simulink model "D_20231120_Modell_Inbetriebnahme_BreakOutBox_Jetson"  (R2022b)
settings: Solver=ode1  StartTime=0.0  StopTime=inf  FixedStep=Ts  RelTol=1e-3
PreLoadFcn:
  | pulsePeriod = 0.05;
  | 
  | Ts = 0.001;
  | 
  | FPGA_Frequency = 75000000;
  | 
  | ts_IO691 = 5e-3;
PostLoadFcn:
  | ewolfSetUp
InitFcn:
  | pulsePeriod = 0.05;
  | 
  | Ts = 0.001;
  | 
  | FPGA_Frequency = 75000000;
  | 
  | ts_IO691 = 5e-3;
StopFcn:
  | Simulink.sdi.clearPreferences;
  | if isfile(['sdi_view_',bdroot,'.mldatx'])
  | Simulink.sdi.view;
  | pause(3);
  | Simulink.sdi.loadView(['sdi_view_',bdroot,]);
  | end
model workspace (MAT data in the model file):
  MaxDreh = 1
values from neighbouring files (symbols this model uses):
  max_ac = 2    [ewolfSetUp.m]
  min_ac = -3    [ewolfSetUp.m]
  PredictionHorizon = 30    [ewolfSetUp.m]
undefined symbols (not defined in the file or in its folder): canChannel, DiscIntNeverNeededParam, Ended, HS, IO291, IO397, max_steer_car, min_steer_car, sigbuilder_block, Single
libraries: lllalib x255, canmsglib x146, simulink x42, speedgoatlib_IO191 x5, speedgoatlib_IO291 x5, slrealtimeiplib x3, speedgoatlib_IO691 x3, slrealtimeutilitieslib x2, spsEdgeDetectorLib x1, simulink_extras x1, speedgoatlib_fpga_dio x1, speedgoatlib_fpga_quadrature x1
(part 2 of 8)

== system D_20231120_Modell_Inbetriebnahme_BreakOutBox_Jetson/Scope ==
  From_Speedgoat : Inport
  To_Speedgoat : Inport  Port=2
  Bus Selector : BusSelector  OutputSignals=IO191_Out.IO191_AI.IO191_AI_CH1_FP_1_G,IO191_Out.IO191_AI.IO191_AI_CH2_FP_2_G,IO191_Out.IO191_AI.IO191_AI_CH3_LG_1_G,IO191_Out.IO191_AI.IO191_AI_CH4_LG_2_G
  Bus Selector1 : BusSelector  OutputSignals=IO691_Out.IO691_CAN_Sensoren.USS,IO691_Out.IO691_CAN_Sensoren.RC_Lenkung,IO691_Out.IO691_CAN_Sensoren.RC_Fahrpedal
  Scope : Scope  NumInputPorts=3
  Scope2 : Scope  NumInputPorts=4
  Terminator : Terminator
  wires:
  Bus Selector/2 -> Scope2/2  "<IO191_AI_CH2_FP_2_G>"
  Bus Selector/1 -> Scope2/1  "<IO191_AI_CH1_FP_1_G>"
  Bus Selector/4 -> Scope2/4  "<IO191_AI_CH4_LG_2_G>"
  From_Speedgoat/1 -> Bus Selector1/1, Bus Selector/1
  Bus Selector/3 -> Scope2/3  "<IO191_AI_CH3_LG_1_G>"
  To_Speedgoat/1 -> Terminator/1
  Bus Selector1/1 -> Scope/1  "<USS>"
  Bus Selector1/2 -> Scope/2  "<RC_Lenkung>"
  Bus Selector1/3 -> Scope/3  "<RC_Fahrpedal>"

== system D_20231120_Modell_Inbetriebnahme_BreakOutBox_Jetson/Bremspedal Steuerung/Moving Average ==
  In : Inport
  Divide : Product  Inputs=*/
  Round : Rounding  Operator=round
  Sum of Elements : Sum  Inputs=+
  Tapped Delay : simulink/Discrete/Tapped Delay  vinit=0.0  samptime=-1  NumDelays=4  DelayOrder=Oldest  includeCurrent=off
  Vector Concatenate : Concatenate
  Width : Width
  Hall_A : Outport
  wires:
  In/1 -> Vector Concatenate/1, Tapped Delay/1
  Sum of Elements/1 -> Divide/1
  Width/1 -> Divide/2
  Vector Concatenate/1 -> Sum of Elements/1, Width/1
  Divide/1 -> Round/1
  Round/1 -> Hall_A/1
  Tapped Delay/1 -> Vector Concatenate/2

== system D_20231120_Modell_Inbetriebnahme_BreakOutBox_Jetson/Bremspedal Steuerung/Moving Average1 ==
  In : Inport
  Divide : Product  Inputs=*/
  Round : Rounding  Operator=round
  Sum of Elements : Sum  Inputs=+
  Tapped Delay : simulink/Discrete/Tapped Delay  vinit=0.0  samptime=-1  NumDelays=4  DelayOrder=Oldest  includeCurrent=off
  Vector Concatenate : Concatenate
  Width : Width
  Hall_B : Outport
  wires:
  In/1 -> Vector Concatenate/1, Tapped Delay/1
  Sum of Elements/1 -> Divide/1
  Width/1 -> Divide/2
  Vector Concatenate/1 -> Sum of Elements/1, Width/1
  Divide/1 -> Round/1
  Round/1 -> Hall_B/1
  Tapped Delay/1 -> Vector Concatenate/2

== system D_20231120_Modell_Inbetriebnahme_BreakOutBox_Jetson/Bremspedal Steuerung/QAD Steuerung ==
  <QAD_Turns> : Inport
  u : Inport  Port=2
  AND : Logic  Inputs=3  AllPortsSameDT=off  OutDataTypeStr=boolean
  AND1 : Logic  AllPortsSameDT=off  OutDataTypeStr=boolean
  AND2 : Logic  AllPortsSameDT=off  OutDataTypeStr=boolean
  Compare To Constant : simulink/Logic and Bit Operations/Compare To Constant  relop=>  const=0.4  OutDataTypeStr=boolean
  Compare To Constant1 : simulink/Logic and Bit Operations/Compare To Constant  relop=<  const=0.1  OutDataTypeStr=boolean
  Compare To Constant2 : simulink/Logic and Bit Operations/Compare To Constant  relop=<  const=0  OutDataTypeStr=boolean
  Compare To Constant3 : simulink/Logic and Bit Operations/Compare To Constant  relop=>=  const=-0.2  OutDataTypeStr=boolean
  Compare To Constant4 : simulink/Logic and Bit Operations/Compare To Constant  relop=<  const=0.9  OutDataTypeStr=boolean
  Compare To Constant5 : simulink/Logic and Bit Operations/Compare To Constant  relop=>  const=0.9  OutDataTypeStr=boolean
  Compare To Constant6 : simulink/Logic and Bit Operations/Compare To Constant  relop=>=  const=-0.4  OutDataTypeStr=boolean
  IC2 : InitialCondition  Value=0
  IC3 : InitialCondition  Value=0
  OR : Logic  Operator=OR  AllPortsSameDT=off  OutDataTypeStr=boolean
  Out1 : Outport
  Out2 : Outport  Port=2
  wires:
  <QAD_Turns>/1 -> Compare To Constant3/1, Compare To Constant2/1, Compare To Constant6/1
  OR/1 -> IC2/1
  AND1/1 -> IC3/1
  IC3/1 -> Out2/1
  u/1 -> Compare To Constant5/1, Compare To Constant4/1, Compare To Constant/1, Compare To Constant1/1
  IC2/1 -> Out1/1
  Compare To Constant/1 -> AND/2
  Compare To Constant6/1 -> AND2/2
  Compare To Constant5/1 -> AND2/1
  AND/1 -> OR/1
  AND2/1 -> OR/2
  Compare To Constant3/1 -> AND/1
  Compare To Constant4/1 -> AND/3
  Compare To Constant1/1 -> AND1/2
  Compare To Constant2/1 -> AND1/1

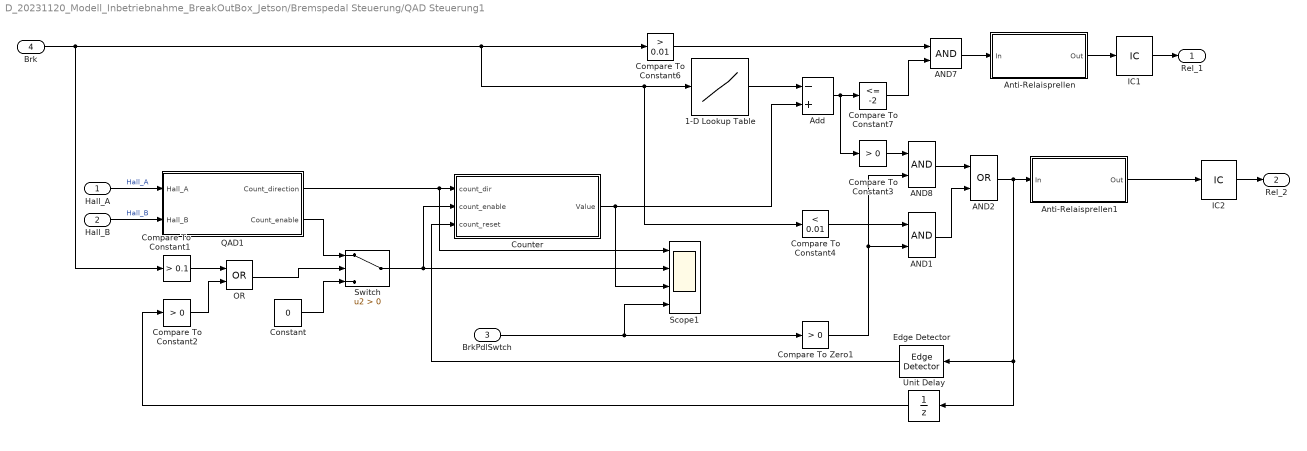
== system D_20231120_Modell_Inbetriebnahme_BreakOutBox_Jetson/Bremspedal Steuerung/QAD Steuerung1 ==
  Hall_A : Inport
  Hall_B : Inport  Port=2
  BrkPdlSwtch : Inport  Port=3
  Brk : Inport  Port=4
  1-D Lookup Table : Lookup_n-D  NumberOfTableDimensions=1  BreakpointsForDimension1=[0, 0.25, 0.5, 0.75, 1]  Table=[0, 10, 20, 30, 80]  InterpMethod=Nearest  InternalRulePriority=Speed  RndMeth=Simplest
  AND1 : Logic  AllPortsSameDT=off  OutDataTypeStr=boolean
  AND2 : Logic  Operator=OR  AllPortsSameDT=off  OutDataTypeStr=boolean
  AND7 : Logic  AllPortsSameDT=off  OutDataTypeStr=boolean
  AND8 : Logic  AllPortsSameDT=off  OutDataTypeStr=boolean
  Add : Sum  Inputs=-+
  Anti-Relaisprellen : Subsystem
  Anti-Relaisprellen1 : Subsystem
  Compare To Constant1 : simulink/Logic and Bit Operations/Compare To Constant  relop=>  const=0.1  OutDataTypeStr=boolean
  Compare To Constant2 : simulink/Logic and Bit Operations/Compare To Constant  relop=>  const=0  OutDataTypeStr=boolean
  Compare To Constant3 : simulink/Logic and Bit Operations/Compare To Constant  relop=>  const=0  OutDataTypeStr=boolean
  Compare To Constant4 : simulink/Logic and Bit Operations/Compare To Constant  relop=<  const=0.01  OutDataTypeStr=boolean
  Compare To Constant6 : simulink/Logic and Bit Operations/Compare To Constant  relop=>  const=0.01  OutDataTypeStr=boolean
  Compare To Constant7 : simulink/Logic and Bit Operations/Compare To Constant  relop=<=  const=-2  OutDataTypeStr=boolean
  Compare To Zero1 : simulink/Logic and Bit Operations/Compare To Zero  relop=>  OutDataTypeStr=boolean
  Constant : Constant  Value=0
  Counter : Subsystem
  Edge Detector : spsEdgeDetectorLib/Edge Detector  model=Falling  ic=0  Ts=0
  IC1 : InitialCondition  Value=0
  IC2 : InitialCondition  Value=0
  OR : Logic  Operator=OR  AllPortsSameDT=off  OutDataTypeStr=boolean
  QAD1 : Subsystem
  Scope1 : Scope  NumInputPorts=4
  Switch : Switch  Criteria=u2 > Threshold  SaturateOnIntegerOverflow=off  InputSameDT=off
  Unit Delay : UnitDelay  SampleTime=-1  HasFrameUpgradeWarning=on
  Rel_1 : Outport
  Rel_2 : Outport  Port=2
  wires:
  Hall_A/1 -> QAD1/1(Hall_A)  "Hall_A"
  Hall_B/1 -> QAD1/2(Hall_B)  "Hall_B"
  QAD1/1(Count_direction) -> Scope1/1, Counter/1(count_dir)
  Compare To Constant6/1 -> AND7/1
  Compare To Constant7/1 -> AND7/2
  Brk/1 -> Compare To Constant1/1, Compare To Constant4/1, 1-D Lookup Table/1, Compare To Constant6/1
  Counter/1(Value) -> Scope1/3, Add/2
  1-D Lookup Table/1 -> Add/1
  Add/1 -> Compare To Constant3/1, Compare To Constant7/1
  Switch/1 -> Counter/2(count_enable), Scope1/2
  AND7/1 -> Anti-Relaisprellen/1(In)
  Anti-Relaisprellen/1(Out) -> IC1/1
  AND2/1 -> Anti-Relaisprellen1/1(In), Edge Detector/1, Unit Delay/1
  Anti-Relaisprellen1/1(Out) -> IC2/1
  BrkPdlSwtch/1 -> Scope1/4, Compare To Zero1/1
  Compare To Zero1/1 -> AND1/2, AND8/2
  Edge Detector/1 -> Counter/3(count_reset)
  Compare To Constant1/1 -> OR/1
  QAD1/2(Count_enable) -> Switch/1
  Constant/1 -> Switch/3
  OR/1 -> Switch/2
  Compare To Constant2/1 -> OR/2
  IC1/1 -> Rel_1/1
  IC2/1 -> Rel_2/1
  Compare To Constant3/1 -> AND8/1
  Unit Delay/1 -> Compare To Constant2/1
  AND8/1 -> AND2/1
  AND1/1 -> AND2/2
  Compare To Constant4/1 -> AND1/1

== system D_20231120_Modell_Inbetriebnahme_BreakOutBox_Jetson/Com Android/Detektion_kein_Signal ==
  In : Inport
  Compare To Constant : simulink/Logic and Bit Operations/Compare To Constant  relop===  const=0  OutDataTypeStr=boolean
  Divide : Product  Inputs=*/
  Sum of Elements : Sum  Inputs=+
  Tapped Delay1 : simulink/Discrete/Tapped Delay  vinit=0.0  samptime=-1  NumDelays=199  DelayOrder=Oldest  includeCurrent=off
  Vector Concatenate : Concatenate
  Width : Width
  Out : Outport  VectorParamsAs1DForOutWhenUnconnected=off
  wires:
  In/1 -> Vector Concatenate/1, Tapped Delay1/1
  Tapped Delay1/1 -> Vector Concatenate/2
  Vector Concatenate/1 -> Sum of Elements/1, Width/1
  Divide/1 -> Compare To Constant/1
  Sum of Elements/1 -> Divide/1
  Width/1 -> Divide/2
  Compare To Constant/1 -> Out/1

== system D_20231120_Modell_Inbetriebnahme_BreakOutBox_Jetson/Com Android/Kurvenanpassung ==
  In1 : Inport
  Add2 : Sum
  Constant6 : Constant  Value=0.5
  Constant7 : Constant  Value=3
  Multiply : Gain  Gain=0.5
  Power : Math  Operator=pow
  Out1 : Outport
  wires:
  Constant6/1 -> Add2/2
  Power/1 -> Multiply/1
  Constant7/1 -> Power/2
  In1/1 -> Power/1
  Add2/1 -> Out1/1
  Multiply/1 -> Add2/1

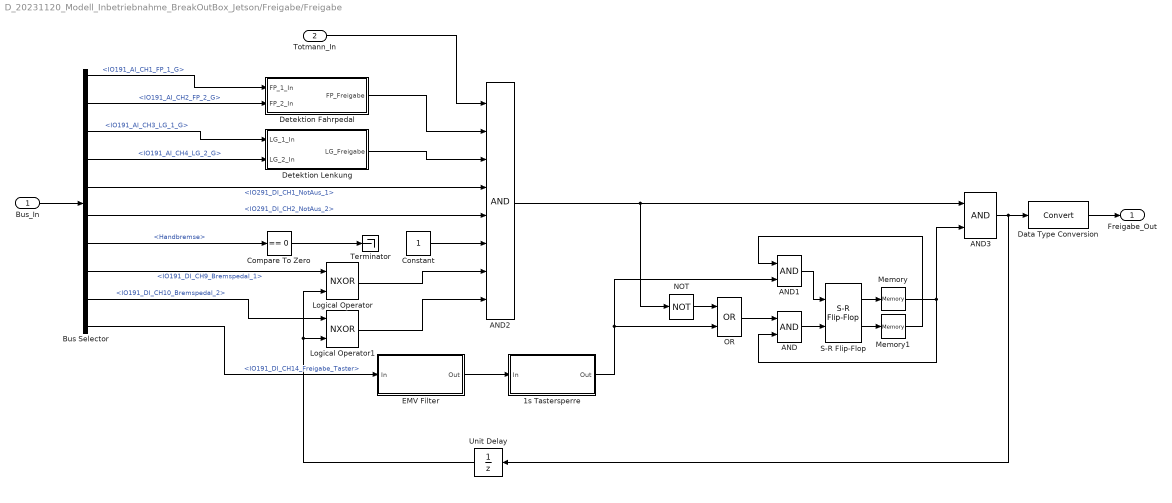
== system D_20231120_Modell_Inbetriebnahme_BreakOutBox_Jetson/Freigabe/Freigabe ==
  Bus_In : Inport
  Totmann_In : Inport  Port=2
  1s Tastersperre : Subsystem
  AND : Logic  AllPortsSameDT=off  OutDataTypeStr=boolean
  AND1 : Logic  AllPortsSameDT=off  OutDataTypeStr=boolean
  AND2 : Logic  Inputs=8  AllPortsSameDT=off  OutDataTypeStr=boolean
  AND3 : Logic  AllPortsSameDT=off  OutDataTypeStr=boolean
  Bus Selector : BusSelector  OutputSignals=IO191_Out.IO191_AI.IO191_AI_CH1_FP_1_G,IO191_Out.IO191_AI.IO191_AI_CH2_FP_2_G,IO191_Out.IO191_AI.IO191_AI_CH3_LG_1_G,IO191_Out.IO191_AI.IO191_AI_CH4_LG_2_G,IO291_Out.IO291_Iso_DI.IO291_DI_CH1_NotAus_1,IO291_Out.IO291_Iso_DI.IO291_DI_CH2_NotAus_2,IO691_Out.IO691_CAN_eWolf.Handbremse,IO191_Out.IO191_DI.IO191_DI_CH9_Bremspedal_1,IO191_Out.IO191_DI.IO191_DI_CH10_Bremspedal_2,IO191_Out.IO191_DI.IO191_DI_CH14_Freigabe_Taster
  Compare To Zero : simulink/Logic and Bit Operations/Compare To Zero  relop===  OutDataTypeStr=boolean
  Constant : Constant
  Data Type Conversion : DataTypeConversion  SaturateOnIntegerOverflow=off  RndMeth=Floor
  Detektion Fahrpedal : Subsystem
  Detektion Lenkung : Subsystem
  EMV Filter : Subsystem
  Logical Operator : Logic  Operator=NXOR  AllPortsSameDT=off  OutDataTypeStr=boolean
  Logical Operator1 : Logic  Operator=NXOR  AllPortsSameDT=off  OutDataTypeStr=boolean
  Memory : Memory  InheritSampleTime=on  LinearizeAsDelay=on
  Memory1 : Memory  InheritSampleTime=on  LinearizeAsDelay=on
  NOT : Logic  Operator=NOT  AllPortsSameDT=off  OutDataTypeStr=boolean
  OR : Logic  Operator=OR  AllPortsSameDT=off  OutDataTypeStr=boolean
  S-R Flip-Flop : simulink_extras/Flip Flops/S-R Flip-Flop  initial_condition=0
  Terminator : Terminator
  Unit Delay : UnitDelay  SampleTime=-1  HasFrameUpgradeWarning=on
  Freigabe_Out : Outport
  wires:
  Bus_In/1 -> Bus Selector/1
  Bus Selector/10 -> EMV Filter/1(In)  "<IO191_DI_CH14_Freigabe_Taster>"
  S-R Flip-Flop/1 -> Memory/1
  AND/1 -> S-R Flip-Flop/2
  S-R Flip-Flop/2 -> Memory1/1
  AND1/1 -> S-R Flip-Flop/1
  Memory/1 -> AND3/2, AND/2
  Data Type Conversion/1 -> Freigabe_Out/1
  Memory1/1 -> AND1/1
  1s Tastersperre/1(Out) -> AND1/2, OR/2
  Totmann_In/1 -> AND2/1
  Bus Selector/1 -> Detektion Fahrpedal/1(FP_1_In)  "<IO191_AI_CH1_FP_1_G>"
  Bus Selector/2 -> Detektion Fahrpedal/2(FP_2_In)  "<IO191_AI_CH2_FP_2_G>"
  Bus Selector/3 -> Detektion Lenkung/1(LG_1_In)  "<IO191_AI_CH3_LG_1_G>"
  Bus Selector/4 -> Detektion Lenkung/2(LG_2_In)  "<IO191_AI_CH4_LG_2_G>"
  Detektion Fahrpedal/1(FP_Freigabe) -> AND2/2
  Detektion Lenkung/1(LG_Freigabe) -> AND2/3
  Bus Selector/5 -> AND2/4  "<IO291_DI_CH1_NotAus_1>"
  Bus Selector/6 -> AND2/5  "<IO291_DI_CH2_NotAus_2>"
  AND2/1 -> NOT/1, AND3/1
  AND3/1 -> Data Type Conversion/1, Unit Delay/1
  OR/1 -> AND/1
  NOT/1 -> OR/1
  Bus Selector/8 -> Logical Operator/1  "<IO191_DI_CH9_Bremspedal_1>"
  Bus Selector/9 -> Logical Operator1/1  "<IO191_DI_CH10_Bremspedal_2>"
  Logical Operator/1 -> AND2/7
  Logical Operator1/1 -> AND2/8
  Unit Delay/1 -> Logical Operator/2, Logical Operator1/2
  EMV Filter/1(Out) -> 1s Tastersperre/1(In)
  Bus Selector/7 -> Compare To Zero/1  "<Handbremse>"
  Compare To Zero/1 -> Terminator/1
  Constant/1 -> AND2/6

== system D_20231120_Modell_Inbetriebnahme_BreakOutBox_Jetson/Freigabe/Totmann ==
  Bus_In : Inport
  AND : Logic  AllPortsSameDT=off  OutDataTypeStr=boolean
  Bus Selector : BusSelector  OutputSignals=IO191_Out.IO191_DI.IO191_DI_CH12_Totmann_Taster_1,IO191_Out.IO191_DI.IO191_DI_CH13_Totmann_Taster_2
  Compare To Constant : simulink/Logic and Bit Operations/Compare To Constant  relop===  const=1  OutDataTypeStr=boolean
  Compare To Constant1 : simulink/Logic and Bit Operations/Compare To Constant  relop===  const=0  OutDataTypeStr=boolean
  Compare To Constant2 : simulink/Logic and Bit Operations/Compare To Constant  relop=<  const=30  OutDataTypeStr=boolean
  Compare To Constant3 : simulink/Logic and Bit Operations/Compare To Constant  relop=<=  const=45  OutDataTypeStr=boolean
  Constant : Constant
  Constant1 : Constant  Value=0
  Constant2 : Constant
  Integrator : Integrator  ExternalReset=rising
  Pulse Generator : DiscretePulseGenerator  PulseType=Time based  PulseWidth=75
  Switch : Switch  Criteria=u2 > Threshold  SaturateOnIntegerOverflow=off  InputSameDT=off
  Switch1 : Switch  Criteria=u2 > Threshold  SaturateOnIntegerOverflow=off  InputSameDT=off
  Switch2 : Switch  Criteria=u2 > Threshold  SaturateOnIntegerOverflow=off  InputSameDT=off
  Totmann_Freigabe : Outport
  Totmann_LED : Outport  Port=2
  wires:
  Bus_In/1 -> Bus Selector/1
  Bus Selector/1 -> Compare To Constant/1  "<IO191_DI_CH12_Totmann_Taster_1>"
  Bus Selector/2 -> Compare To Constant1/1  "<IO191_DI_CH13_Totmann_Taster_2>"
  Compare To Constant/1 -> AND/1
  Compare To Constant1/1 -> AND/2
  Constant/1 -> Switch/1, Integrator/1
  AND/1 -> Integrator/2
  Switch/1 -> Switch1/1
  Integrator/1 -> Compare To Constant3/1, Compare To Constant2/1
  Compare To Constant2/1 -> Switch/2
  Pulse Generator/1 -> Switch/3
  Switch1/1 -> Totmann_LED/1
  Compare To Constant3/1 -> Switch2/2, Switch1/2
  Constant1/1 -> Switch2/3, Switch1/3
  Switch2/1 -> Totmann_Freigabe/1
  Constant2/1 -> Switch2/1

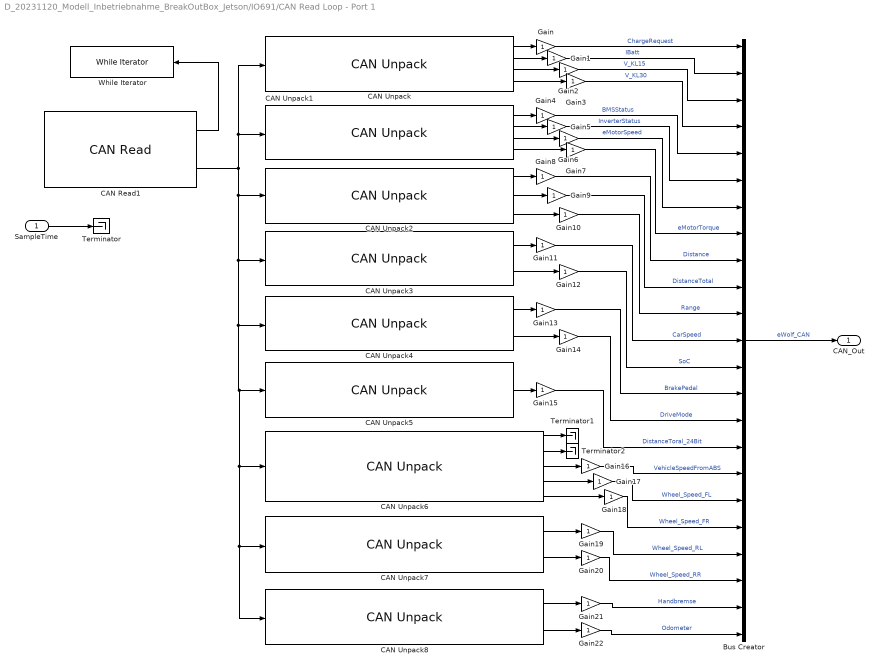
== system D_20231120_Modell_Inbetriebnahme_BreakOutBox_Jetson/IO691/CAN Read Loop - Port 1 ==
  SampleTime : Inport
  Bus Creator : BusCreator  Inputs=23
  CAN Read1 : speedgoatlib_IO691/Legacy/CAN Read  id=1  ts=-1  channel=2  messageType=CAN  canType=CAN (HS)  BusOutput=off  initValues=[691 1 -1 1 1 1 0]
      settings: SourceProductName=Simulink Real-Time: Speedgoat I/O Blockset
  CAN Unpack : canmsglib/CAN Unpack  CANdbFile=eWolf_FZG_V2.dbc  MsgList=VCU2DL2  MsgName=VCU2DL2  MsgIDType=Standard (11-bit identifier)  MsgIdentifier=1041  MsgLength=8  SignalInfo={'ChargeRequest','56','16','BE','unsigned','Standard','0','0.01','0','0','655.35';'IBatt','8','16','BE','signed','Standard','0','0.01','0','-32767','32768';'V_KL15','40','16','BE','unsigned','Standard','0','0.01','0','0','65535';'V_KL30','24','16','BE','unsigned','Standard','0','0.01','0','0','65535'}  IDPort=off  TimestampPort=off  ErrorPort=off  RemotePort=off  LengthPort=off  StatusPort=off  ApplyMinMax=off
      settings: DataFormat=CANdb specified signals
  CAN Unpack1 : canmsglib/CAN Unpack  CANdbFile=eWolf_FZG_V2.dbc  MsgList=VCU2DL3  MsgName=VCU2DL3  MsgIDType=Standard (11-bit identifier)  MsgIdentifier=1045  MsgLength=8  SignalInfo={'BMSStatus','56','16','BE','unsigned','Standard','0','1','0','0','65535';'InverterStatus','40','16','BE','unsigned','Standard','0','1','0','0','65535';'eMotorSpeed','24','16','BE','signed','Standard','0','0.01','0','-32767','32768';'eMotorTorque','8','16','BE','signed','Standard','0','0.01','0','-32767','32768'}  IDPort=off  TimestampPort=off  ErrorPort=off  RemotePort=off  LengthPort=off  StatusPort=off  ApplyMinMax=off
      settings: DataFormat=CANdb specified signals
  CAN Unpack2 : canmsglib/CAN Unpack  CANdbFile=eWolf_FZG_V2.dbc  MsgList=VCU2DL4  MsgName=VCU2DL4  MsgIDType=Standard (11-bit identifier)  MsgIdentifier=1056  MsgLength=8  SignalInfo={'Distance','24','16','BE','unsigned','Standard','0','0.1','0','0','65535';'DistanceTotal','56','32','BE','unsigned','Standard','0','0.1','0','0','429496729.5';'Range','8','16','BE','unsigned','Standard','0','0.1','0','0','65535'}  IDPort=off  TimestampPort=off  ErrorPort=off  RemotePort=off  LengthPort=off  StatusPort=off  ApplyMinMax=off
      settings: DataFormat=CANdb specified signals
  CAN Unpack3 : canmsglib/CAN Unpack  CANdbFile=eWolf_FZG_V2.dbc  MsgList=VCU2DL5  MsgName=VCU2DL5  MsgIDType=Standard (11-bit identifier)  MsgIdentifier=1057  MsgLength=8  SignalInfo={'CarSpeed','16','16','BE','unsigned','Standard','0','0.1','0','0','65535';'SoC','0','8','BE','unsigned','Standard','0','0.5','0','0','255'}  IDPort=off  TimestampPort=off  ErrorPort=off  RemotePort=off  LengthPort=off  StatusPort=off  ApplyMinMax=off
      settings: DataFormat=CANdb specified signals
  CAN Unpack4 : canmsglib/CAN Unpack  CANdbFile=eWolf_FZG_V2.dbc  MsgList=VCU2DL7  MsgName=VCU2DL7  MsgIDType=Standard (11-bit identifier)  MsgIdentifier=1059  MsgLength=8  SignalInfo={'BrakePedal','8','1','BE','unsigned','Standard','0','1','0','0','1';'DriveMode','0','8','BE','unsigned','Standard','0','1','0','0','255'}  IDPort=off  TimestampPort=off  ErrorPort=off  RemotePort=off  LengthPort=off  StatusPort=off  ApplyMinMax=off
      settings: DataFormat=CANdb specified signals
  CAN Unpack5 : canmsglib/CAN Unpack  CANdbFile=eWolf_FZG_V2.dbc  MsgList=VCU_0x400  MsgName=VCU_0x400  MsgIDType=Standard (11-bit identifier)  MsgIdentifier=1024  MsgLength=8  SignalInfo={'DistanceTotal_24Bit','56','24','BE','unsigned','Standard','0','1','0','0','16777215'}  IDPort=off  TimestampPort=off  ErrorPort=off  RemotePort=off  LengthPort=off  StatusPort=off  ApplyMinMax=off
      settings: DataFormat=CANdb specified signals
  CAN Unpack6 : canmsglib/CAN Unpack  CANdbFile=eWolf_FZG_V2.dbc  MsgList=Wheel_Speed_Front  MsgName=Wheel_Speed_Front  MsgIDType=Standard (11-bit identifier)  MsgIdentifier=644  MsgLength=8  SignalInfo={'DistanceTraveled1','48','8','LE','signed','Standard','0','1','0','-Inf','Inf';'DistanceTraveled2','56','8','LE','signed','Standard','0','1','0','-Inf','Inf';'VehicleSpeedFromABS','40','16','BE','unsigned','Standard','0','1','0','-Inf','Inf';'Wheel_Speed_FL','24','16','BE','unsigned','Standard','0','0.005','0','0','327';'Wheel_Speed_FR','8','16','BE','unsigned','Standard','0','0.005','0','0','327'}  IDPort=off  TimestampPort=off  ErrorPort=off  RemotePort=off  LengthPort=off  StatusPort=off  ApplyMinMax=off
      settings: DataFormat=CANdb specified signals
  CAN Unpack7 : canmsglib/CAN Unpack  CANdbFile=eWolf_FZG_V2.dbc  MsgList=Wheel_Speed_Rear  MsgName=Wheel_Speed_Rear  MsgIDType=Standard (11-bit identifier)  MsgIdentifier=645  MsgLength=8  SignalInfo={'Wheel_Speed_RL','24','16','BE','unsigned','Standard','0','0.005','0','0','327';'Wheel_Speed_RR','8','16','BE','unsigned','Standard','0','0.005','0','0','327'}  IDPort=off  TimestampPort=off  ErrorPort=off  RemotePort=off  LengthPort=off  StatusPort=off  ApplyMinMax=off
      settings: DataFormat=CANdb specified signals
  CAN Unpack8 : canmsglib/CAN Unpack  CANdbFile=eWolf_FZG_V2.dbc  MsgList=Bremse_Odo  MsgName=Bremse_Odo  MsgIDType=Standard (11-bit identifier)  MsgIdentifier=1477  MsgLength=8  SignalInfo={'Handbremse','2','1','LE','unsigned','Standard','0','1','0','-Inf','Inf';'Odometer','24','24','BE','unsigned','Standard','0','1','-1937','-1937','16775278'}  IDPort=off  TimestampPort=off  ErrorPort=off  RemotePort=off  LengthPort=off  StatusPort=off  ApplyMinMax=off
      settings: DataFormat=CANdb specified signals
  Gain{,1..22} (23 alike) : Gain
  Terminator : Terminator
  Terminator1 : Terminator
  Terminator2 : Terminator
  While Iterator : WhileIterator  MaxIters=501  WhileBlockType=do-while
  CAN_Out : Outport
  wires:
  SampleTime/1 -> Terminator/1
  CAN Read1/1 -> While Iterator/1
  CAN Read1/2 -> CAN Unpack8/1, CAN Unpack7/1, CAN Unpack6/1, CAN Unpack5/1, CAN Unpack4/1, CAN Unpack3/1, CAN Unpack2/1, CAN Unpack1/1, CAN Unpack/1
  CAN Unpack/1 -> Gain/1
  CAN Unpack/2 -> Gain1/1
  CAN Unpack/3 -> Gain2/1
  CAN Unpack/4 -> Gain3/1
  CAN Unpack1/1 -> Gain4/1
  CAN Unpack1/2 -> Gain5/1
  CAN Unpack1/3 -> Gain6/1
  CAN Unpack1/4 -> Gain7/1
  CAN Unpack2/1 -> Gain8/1
  CAN Unpack2/2 -> Gain9/1
  CAN Unpack2/3 -> Gain10/1
  CAN Unpack3/1 -> Gain11/1
  CAN Unpack3/2 -> Gain12/1
  CAN Unpack4/1 -> Gain13/1
  CAN Unpack4/2 -> Gain14/1
  CAN Unpack5/1 -> Gain15/1
  Gain/1 -> Bus Creator/1  "ChargeRequest"
  Gain1/1 -> Bus Creator/2  "IBatt"
  Gain2/1 -> Bus Creator/3  "V_KL15"
  Gain3/1 -> Bus Creator/4  "V_KL30"
  Gain4/1 -> Bus Creator/5  "BMSStatus"
  Gain5/1 -> Bus Creator/6  "InverterStatus"
  Gain6/1 -> Bus Creator/7  "eMotorSpeed"
  Gain7/1 -> Bus Creator/8  "eMotorTorque"
  Gain8/1 -> Bus Creator/9  "Distance"
  Gain9/1 -> Bus Creator/10  "DistanceTotal"
  Gain10/1 -> Bus Creator/11  "Range"
  Gain11/1 -> Bus Creator/12  "CarSpeed"
  Gain12/1 -> Bus Creator/13  "SoC"
  Gain13/1 -> Bus Creator/14  "BrakePedal"
  Gain14/1 -> Bus Creator/15  "DriveMode"
  Gain15/1 -> Bus Creator/16  "DistanceToral_24Bit"
  Bus Creator/1 -> CAN_Out/1  "eWolf_CAN"
  CAN Unpack6/1 -> Terminator1/1
  CAN Unpack6/2 -> Terminator2/1
  CAN Unpack6/3 -> Gain16/1
  CAN Unpack6/4 -> Gain17/1
  CAN Unpack6/5 -> Gain18/1
  Gain16/1 -> Bus Creator/17  "VehicleSpeedFromABS"
  Gain17/1 -> Bus Creator/18  "Wheel_Speed_FL"
  Gain18/1 -> Bus Creator/19  "Wheel_Speed_FR"
  CAN Unpack7/1 -> Gain19/1
  CAN Unpack7/2 -> Gain20/1
  Gain19/1 -> Bus Creator/20  "Wheel_Speed_RL"
  Gain20/1 -> Bus Creator/21  "Wheel_Speed_RR"
  CAN Unpack8/1 -> Gain21/1
  CAN Unpack8/2 -> Gain22/1
  Gain21/1 -> Bus Creator/22  "Handbremse"
  Gain22/1 -> Bus Creator/23  "Odometer"

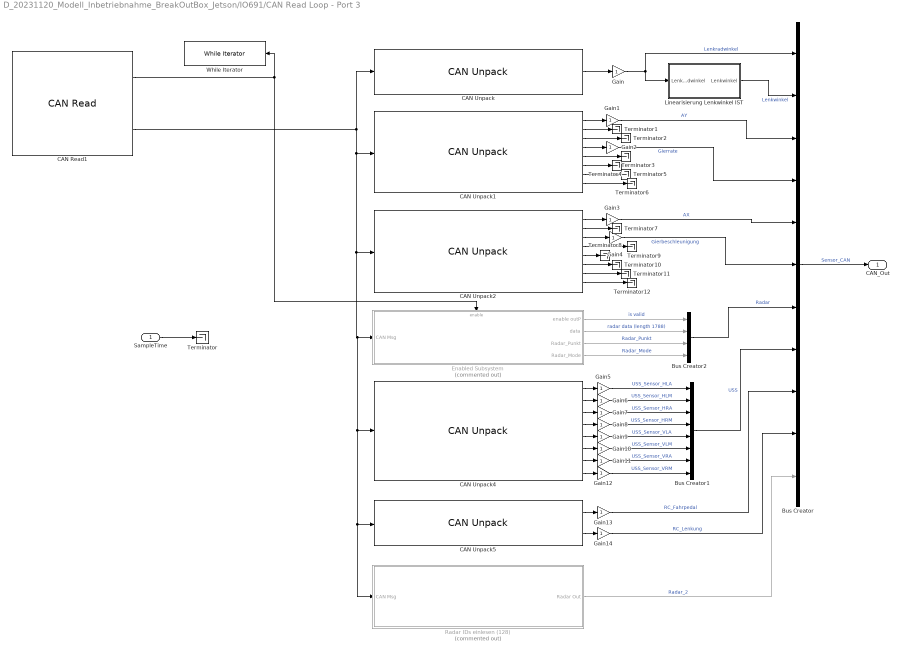
== system D_20231120_Modell_Inbetriebnahme_BreakOutBox_Jetson/IO691/CAN Read Loop - Port 3 ==
  SampleTime : Inport
  Bus Creator : BusCreator  Inputs=11
  Bus Creator1 : BusCreator  Inputs=8
  Bus Creator2 : BusCreator  Inputs=4
  CAN Read1 : speedgoatlib_IO691/Legacy/CAN Read  id=1  ts=-1  channel=1  messageType=CAN  canType=CAN (HS)  BusOutput=off  initValues=[691 1 -1 0 1 1 0]
      settings: SourceProductName=Simulink Real-Time: Speedgoat I/O Blockset
  CAN Unpack : canmsglib/CAN Unpack  CANdbFile=eWolf_SensorCAN.dbc  MsgList=Lenkwinkelsensor  MsgName=Lenkwinkelsensor  MsgIDType=Standard (11-bit identifier)  MsgIdentifier=2  MsgLength=5  SignalInfo={'Lenkwinkel','0','16','LE','signed','Standard','0','0.09882','0','-630','630'}  IDPort=off  TimestampPort=off  ErrorPort=off  RemotePort=off  LengthPort=off  StatusPort=off  ApplyMinMax=off
      settings: DataFormat=CANdb specified signals
  CAN Unpack1 : canmsglib/CAN Unpack  CANdbFile=eWolf_SensorCAN.dbc  MsgList=Beschleunigungssensor  MsgName=Beschleunigungssensor  MsgIDType=Standard (11-bit identifier)  MsgIdentifier=304  MsgLength=8  SignalInfo={'AY1','32','16','LE','unsigned','Standard','0','0.0001274','-4.1768','-4.1768','4.1768';'AY1_STAT','48','4','LE','unsigned','Standard','0','1','0','0','15';'CLU_STAT','16','4','LE','unsigned','Standard','0','1','0','0','15';'Gierrate','0','16','LE','unsigned','Standard','0','0.005','-163.84','-163.84','163.84';'Gierrate_STAT','52','4','LE','unsigned','Standard','0','1','0','0','15';'PSIP1_EXT_STAT','24','8','LE','unsigned','Standard','0','1','0','0','255';'TX1_CRC','56','8','LE','unsigned','Standard','0','1','0','0','255';'TX1_MSG_CNT','20','4','LE','unsigned','Standard','0','1','0','0','15'}  IDPort=off  TimestampPort=off  ErrorPort=off  RemotePort=off  LengthPort=off  StatusPort=off  ApplyMinMax=off
      settings: DataFormat=CANdb specified signals
  CAN Unpack2 : canmsglib/CAN Unpack  CANdbFile=eWolf_SensorCAN.dbc  MsgList=Beschleunigungssensor_2  MsgName=Beschleunigungssensor_2  MsgIDType=Standard (11-bit identifier)  MsgIdentifier=305  MsgLength=8  SignalInfo={'AX1','32','16','LE','unsigned','Standard','0','0.0001274','-4.1768','-4.1768','4.1768';'AX1_STAT','52','4','LE','unsigned','Standard','0','1','0','0','15';'Gierbeschleunigung','0','16','LE','unsigned','Standard','0','0.125','-4096','-4096','4096';'Gierbeschleunigung_STAT','20','4','LE','unsigned','Standard','0','1','0','0','15';'TX2_CRC','56','8','LE','unsigned','Standard','0','1','0','0','255';'TX2_MSG_CNT','48','4','LE','unsigned','Standard','0','1','0','0','15';'TX2_RES1','16','4','LE','unsigned','Standard','0','1','0','0','15';'TX2_RES2','24','8','LE','unsigned','Standard','0','1','0','0','255'}  IDPort=off  TimestampPort=off  ErrorPort=off  RemotePort=off  LengthPort=off  StatusPort=off  ApplyMinMax=off
      settings: DataFormat=CANdb specified signals
  CAN Unpack4 : canmsglib/CAN Unpack  CANdbFile=eWolf_SensorCAN.dbc  MsgList=Ultraschallsystem  MsgName=Ultraschallsystem  MsgIDType=Standard (11-bit identifier)  MsgIdentifier=16  MsgLength=8  SignalInfo={'USS_Sensor_HLA','32','8','LE','unsigned','Standard','0','1','0','0','255';'USS_Sensor_HLM','40','8','LE','unsigned','Standard','0','1','0','0','255';'USS_Sensor_HRA','56','8','LE','unsigned','Standard','0','1','0','0','255';'USS_Sensor_HRM','48','8','LE','unsigned','Standard','0','1','0','0','255';'USS_Sensor_VLA','0','8','LE','unsigned','Standard','0','1','0','0','255';'USS_Sensor_VLM','8','8','LE','unsigned','Standard','0','1','0','0','255';'USS_Sensor_VRA','24','8','LE','unsigned','Standard','0','1','0','0','255';'USS_Sensor_VRM','16','8','LE','unsigned','Standard','0','1','0','0','255'}  IDPort=off  TimestampPort=off  ErrorPort=off  RemotePort=off  LengthPort=off  StatusPort=off  ApplyMinMax=off
      settings: DataFormat=CANdb specified signals
  CAN Unpack5 : canmsglib/CAN Unpack  CANdbFile=eWolf_SensorCAN.dbc  MsgList=RC_Fernsteuerung  MsgName=RC_Fernsteuerung  MsgIDType=Standard (11-bit identifier)  MsgIdentifier=17  MsgLength=2  SignalInfo={'RC_Fahrpedal','8','8','LE','unsigned','Standard','0','1','0','0','255';'RC_Lenkung','0','8','LE','unsigned','Standard','0','1','0','0','255'}  IDPort=off  TimestampPort=off  ErrorPort=off  RemotePort=off  LengthPort=off  StatusPort=off  ApplyMinMax=off
      settings: DataFormat=CANdb specified signals
  Enabled Subsystem : Subsystem  Commented=on  TreatAsAtomicUnit=on
  Gain{,1..14} (15 alike) : Gain
  Linearisierung Lenkwinkel IST : Subsystem
  Radar IDs einlesen (128) : Subsystem  Commented=on
  Terminator{,1..12} (13 alike) : Terminator
  While Iterator : WhileIterator  MaxIters=501  WhileBlockType=do-while
  CAN_Out : Outport
  wires:
  SampleTime/1 -> Terminator/1
  CAN Read1/1 -> Enabled Subsystem/Enable, While Iterator/1
  CAN Read1/2 -> CAN Unpack/1, Radar IDs einlesen (128)/1(CAN Msg), CAN Unpack5/1, CAN Unpack4/1, Enabled Subsystem/1(CAN Msg), CAN Unpack2/1, CAN Unpack1/1
  Bus Creator/1 -> CAN_Out/1  "Sensor_CAN"
  CAN Unpack1/1 -> Gain1/1
  CAN Unpack1/5 -> Terminator3/1
  CAN Unpack2/1 -> Gain3/1
  CAN Unpack2/5 -> Terminator8/1
  CAN Unpack1/2 -> Terminator1/1
  CAN Unpack1/3 -> Terminator2/1
  CAN Unpack1/4 -> Gain2/1
  CAN Unpack1/6 -> Terminator4/1
  CAN Unpack1/7 -> Terminator5/1
  CAN Unpack1/8 -> Terminator6/1
  Gain/1 -> Linearisierung Lenkwinkel IST/1(Lenkradwinkel), Bus Creator/1  "Lenkradwinkel"
  Gain1/1 -> Bus Creator/3  "AY"
  Gain2/1 -> Bus Creator/4  "Gierrate"
  Gain3/1 -> Bus Creator/5  "AX"
  Gain4/1 -> Bus Creator/6  "Gierbeschleunigung"
  CAN Unpack2/2 -> Terminator7/1
  CAN Unpack2/3 -> Gain4/1
  CAN Unpack2/4 -> Terminator9/1
  CAN Unpack2/6 -> Terminator10/1
  CAN Unpack2/7 -> Terminator11/1
  CAN Unpack2/8 -> Terminator12/1
  CAN Unpack4/1 -> Gain5/1
  CAN Unpack4/2 -> Gain6/1
  CAN Unpack4/3 -> Gain7/1
  CAN Unpack4/4 -> Gain8/1
  CAN Unpack4/5 -> Gain9/1
  CAN Unpack4/6 -> Gain10/1
  CAN Unpack4/7 -> Gain11/1
  CAN Unpack4/8 -> Gain12/1
  Gain5/1 -> Bus Creator1/1  "USS_Sensor_HLA"
  Gain6/1 -> Bus Creator1/2  "USS_Sensor_HLM"
  Gain7/1 -> Bus Creator1/3  "USS_Sensor_HRA"
  Gain8/1 -> Bus Creator1/4  "USS_Sensor_HRM"
  Gain9/1 -> Bus Creator1/5  "USS_Sensor_VLA"
  Gain10/1 -> Bus Creator1/6  "USS_Sensor_VLM"
  Gain11/1 -> Bus Creator1/7  "USS_Sensor_VRA"
  Gain12/1 -> Bus Creator1/8  "USS_Sensor_VRM"
  Bus Creator1/1 -> Bus Creator/8  "USS"
  CAN Unpack5/1 -> Gain13/1
  CAN Unpack5/2 -> Gain14/1
  Gain13/1 -> Bus Creator/9  "RC_Fahrpedal"
  Gain14/1 -> Bus Creator/10  "RC_Lenkung"
  Enabled Subsystem/1(enable outP) -> Bus Creator2/1  "is valid"
  Enabled Subsystem/2(data) -> Bus Creator2/2  "radar data (length 1788)"
  Enabled Subsystem/3(Radar_Punkt) -> Bus Creator2/3  "Radar_Punkt"
  Enabled Subsystem/4(Radar_Mode) -> Bus Creator2/4  "Radar_Mode"
  Bus Creator2/1 -> Bus Creator/7  "Radar"
  Radar IDs einlesen (128)/1(Radar Out) -> Bus Creator/11  "Radar_2"
  CAN Unpack/1 -> Gain/1
  Linearisierung Lenkwinkel IST/1(Lenkwinkel) -> Bus Creator/2  "Lenkwinkel"

== system D_20231120_Modell_Inbetriebnahme_BreakOutBox_Jetson/Lenkung Steuerung/Beobachter und Begrenzer ==
  note: LwnkungsBeobachter
  note: Lenkwinkelbegrenzung und Lenkdrehmomentbegrenzer
  <CarSpeed> : Inport
  <Lenkwinkel> : Inport  Port=2
  IST Lenkwinkel : Inport  Port=3
  Drehmomvor. norm. : Inport  Port=4
  Lenkwingelgeschwindigkeitsbegrenzer : Subsystem
  Lenkwinkelbegrenzer : Subsystem
  Subsystem1 : Subsystem
  Drehmoment norm. begr. : Outport
  wires:
  Subsystem1/1(lenkradwinkelMaxNomiert) -> Lenkwinkelbegrenzer/3("Maximaler Lenkwinkel normiert und Geschwindigkeitsabhängig ")
  Lenkwinkelbegrenzer/1("Drehmomvor. norm. ") -> Lenkwingelgeschwindigkeitsbegrenzer/1("Drehmomvor. norm. ")
  Subsystem1/2(LenkDrehmomentMaxNomiert) -> Lenkwingelgeschwindigkeitsbegrenzer/2(LenkDrehmomentMaxNomiert)
  <CarSpeed>/1 -> Subsystem1/1(Geschwindigkeit)
  IST Lenkwinkel/1 -> Lenkwinkelbegrenzer/1(Lenkwinkel nomiert)
  Lenkwingelgeschwindigkeitsbegrenzer/1(Drehmoment norm. begr.) -> Drehmoment norm. begr./1
  Drehmomvor. norm./1 -> Lenkwinkelbegrenzer/2(Drehmomvor. norm.)
  <Lenkwinkel>/1 -> Subsystem1/2(Lenkwinkel)

== system D_20231120_Modell_Inbetriebnahme_BreakOutBox_Jetson/Lenkung Steuerung/Lenkmomentsimulationssignalgeber ==
  1-D Lookup Table : Lookup_n-D  NumberOfTableDimensions=1  BreakpointsForDimension1=[min_steer_car max_steer_car]  Table=[1 0]  InternalRulePriority=Speed  RndMeth=Simplest
  Constant3 : Constant
  From File : FromFile  FileName=JetsonTrajektorie2.mat  SampleTime=0
  Index Vector2 : MultiPortSwitch  DataPortOrder=Zero-based contiguous  Inputs=6  zeroidx=on  SaturateOnIntegerOverflow=off  InputSameDT=off
  Rotary Switch3 : RotarySwitchBlock
      settings: Values={{'Jetson', 'Signal 1', 'Signal 2', 'Signal 3', 'Signal 4', 'Signal 5'}, [0 1 2 3 4 5]}
  Saturation : Saturate  UpperLimit=1  LowerLimit=0
  Signal Builder : Subsystem  Tag=STV Subsys  LoadFcn=sigbuilder_block('load');  StartFcn=sigbuilder_block('start');  StopFcn=sigbuilder_block('stop');  ClipboardFcn=sigbuilder_block('clipboard');  mask(Sigbuilder block){tuvar=[0:10]}
      mask help: Simulink:masks:SigbuilderBlock_MD
      mask init:
      | if ~strcmp(get_param(bdroot(gcbh),'SimulationStatus'),'stopped') tuvar = sigbuilder_block('maskInit'); end
      settings: CopyFcn=sigbuilder_block('copy');  DeleteFcn=sigbuilder_block('delete');  ModelCloseFcn=sigbuilder_block('modelClose');  PreSaveFcn=sigbuilder_block('preSave');  PauseFcn=sigbuilder_block('pause');  ContinueFcn=sigbuilder_block('continue');  NameChangeFcn=sigbuilder_block('namechange');  OpenFcn=sigbuilder_block('open',[5.4 36 1141.2 516.6 ]);  CloseFcn=sigbuilder_block('close');
      mask Display: plot(0, 0, 100, 100,[2, 2, 32, 32, 2], [68, 8, 8, 68, 68],[32, 2], [38, 38], [32, 19, 2],[53, 60, 44], [32, 17, 17, 2],[16, 16, 31, 31]);txt = getActiveGroup(gcbh);text(2, 100, txt,'verticalAlignment', 'top');
  Sim_LenkwinkelSoll : Outport
  wires:
  Constant3/1 -> Index Vector2/1
  Signal Builder/1(Signal 1) -> Index Vector2/3
  Signal Builder/2(Signal 2) -> Index Vector2/4
  Signal Builder/3(Signal 3) -> Index Vector2/5
  Signal Builder/4(Signal 4) -> Index Vector2/6
  Index Vector2/1 -> 1-D Lookup Table/1
  Signal Builder/5(Signal 5) -> Index Vector2/7
  1-D Lookup Table/1 -> Saturation/1
  Saturation/1 -> Sim_LenkwinkelSoll/1
  From File/1 -> Index Vector2/2  "LenkwinkelVorgabeMessungJetson"

== system D_20231120_Modell_Inbetriebnahme_BreakOutBox_Jetson/Lenkung Steuerung/Linearisierung Lenkmoment Jetson ==
  <steering_angle> : Inport
  1-D Lookup Table2 : Lookup_n-D  NumberOfTableDimensions=1  BreakpointsForDimension1=[min_steer_car max_steer_car]  Table=[0 1]  InternalRulePriority=Speed  RndMeth=Simplest
  Lenkung umdrehen : Gain  Gain=-1
  Saturation1 : Saturate  UpperLimit=1  LowerLimit=0
  Umrechnen von rad in grad : Gain  Gain=180/pi
  Jetson_LenkwinkelSoll : Outport
  wires:
  <steering_angle>/1 -> Lenkung umdrehen/1
  Saturation1/1 -> Jetson_LenkwinkelSoll/1
  Lenkung umdrehen/1 -> Umrechnen von rad in grad/1  "JetsonWinkelRad"
  Umrechnen von rad in grad/1 -> 1-D Lookup Table2/1  "JetsonWinkelGrad"
  1-D Lookup Table2/1 -> Saturation1/1  "JetsonWinkelGradNormiert"

== system D_20231120_Modell_Inbetriebnahme_BreakOutBox_Jetson/Lenkung Steuerung/Linearisierung Lenkwinkel IST ==
  <Lenkwinkel> : Inport
  1-D Lookup Table : Lookup_n-D  NumberOfTableDimensions=1  BreakpointsForDimension1=[min_steer_car max_steer_car]  Table=[1 0]  InternalRulePriority=Speed  RndMeth=Simplest
  Saturation : Saturate  UpperLimit=1  LowerLimit=0
  Lenkwinkel normiert : Outport
  wires:
  <Lenkwinkel>/1 -> 1-D Lookup Table/1
  Saturation/1 -> Lenkwinkel normiert/1
  1-D Lookup Table/1 -> Saturation/1

== system D_20231120_Modell_Inbetriebnahme_BreakOutBox_Jetson/Lenkung Steuerung/Regler ==
  note: Ausschalten der Regelabweichung
      | bei nicht vorhandener Freigabe
  "Ist " : Inport
  Freigabe : Inport  Port=2
  Soll : Inport  Port=3
  1-D Lookup Table4 : Lookup_n-D  NumberOfTableDimensions=1  BreakpointsForDimension1=[-1 -0.0001 0.0001 1]  Table=[-1.13 -0.13 0.13 1.13]  InternalRulePriority=Speed  RndMeth=Simplest
  Constant : Constant  Value=0.5
  Constant1 : Constant  Value=0.3
  Constant5 : Constant  Value=10
  Constant6 : Constant  Value=0
  Gain : Gain  Gain=-1
  Gain1 : Gain  Gain=-1
  PID Controller : slpidlib/PID Controller  Controller=PI  Form=Parallel  TimeDomain=Continuous-time  UseExternalTs=off  SampleTime=-1  IntegratorMethod=Forward Euler  FilterMethod=Forward Euler  ControllerParametersSource=external  P=2.5  I=1  UseKiTs=off  D=1  N=1  UseFilter=on  TunerSelectOption=Transfer Function Based (PID Tuner App)  InitialConditionSource=internal  InitialConditionForIntegrator=0  InitialConditionForFilter=0  DifferentiatorICPrevScaledInput=0  ExternalReset=level  TrackingMode=off  Kt=1  LimitOutput=on  SatLimitsSource=internal  UpperSaturationLimit=0.5  LowerSaturationLimit=-0.5  LinearizeAsGain=on  AntiWindupMode=none  Kb=1  LimitIntegrator=off  UpperIntegratorSaturationLimit=inf  LowerIntegratorSaturationLimit=-inf  POutMin=[]  POutMax=[]  IOutMin=[]  IOutMax=[]  DOutMin=[]  DOutMax=[]  NOutMin=[]  NOutMax=[]  SumOutMin=[]  SumOutMax=[]  SaturationOutMin=[]  SaturationOutMax=[]  PParamMin=[]  PParamMax=[]  IParamMin=[]  IParamMax=[]  DParamMin=[]  DParamMax=[]  NParamMin=[]  NParamMax=[]  KbParamMin=[]  KbParamMax=[]  KtParamMin=[]  KtParamMax=[]  KbOutMin=[]  KbOutMax=[]  KtOutMin=[]  KtOutMax=[]  IntegratorOutMin=[]  IntegratorOutMax=[]  FilterOutMin=[]  FilterOutMax=[]  SumI1OutMin=[]  SumI1OutMax=[]  SumI2OutMin=[]  SumI2OutMax=[]  SumI3OutMin=[]  SumI3OutMax=[]  SumI4OutMin=[]  SumI4OutMax=[]  SumDOutMin=[]  SumDOutMax=[]  DifferentiatorOutMin=[]  DifferentiatorOutMax=[]  FilterDiffOutCoefMin=[]  FilterDiffOutCoefMax=[]  ReciprocalOutMin=[]  ReciprocalOutMax=[]  SumDenOutMin=[]  SumDenOutMax=[]  SumNumOutMin=[]  SumNumOutMax=[]  DivideOutMin=[]  DivideOutMax=[]  UdiffTsProdOutMin=[]  UdiffTsProdOutMax=[]  NTsProdOutMin=[]  NTsProdOutMax=[]  UintegralTsProdOutMin=[]  UintegralTsProdOutMax=[]  UngainTsProdOutMin=[]  UngainTsProdOutMax=[]  ClampingZeroOutDataTypeStr=Inherit: Inherit via back propagation  ClampingZeroOutMin=[]  ClampingZeroOutMax=[]  FilterDenConstantOutDataTypeStr=Inherit: Inherit via back propagation  FilterDenConstantOutMin=[]  FilterDenConstantOutMax=[]  PCopyOutDataTypeStr=Inherit: Inherit via back propagation  PCopyOutMin=[]  PCopyOutMax=[]  NCopyOutDataTypeStr=Inherit: Inherit via back propagation  NCopyOutMin=[]  NCopyOutMax=[]  IntegratorContinuousStateAttributes=''  IntegratorStateMustResolveToSignalObject=off  IntegratorRTWStateStorageClass=Auto  FilterContinuousStateAttributes=''  FilterStateMustResolveToSignalObject=off  FilterRTWStateStorageClass=Auto  ParallelPVariant=ExternalParameters  IdealPVariant=Disabled  IVariant=ExternalParameters  DVariant=Disabled  IntegratorVariant=Continuous  SatVariant=Enabled  AWVariant=Passthrough  PCopyVariant=Disabled  TRVariant=Disabled  FdbkBlocksVariant=Forward  IdealPFdbkVariant=Disabled  SatFdbkVariant=Disabled  DerivativeFilterVariant=Disabled  NVariant=Disabled  NCopyVariant=Disabled_SignalSpec  FilterICVariant=Disabled  IntegratorICVariant=InternalICs  ExternalResetVariant=ExternalReset  TRSumVariant=Passthrough  SumFdbkVariant=Disabled  SumVariant=Sum_PI  TsampFilterVariant=InternalTs  TsampNgainVariant=Passthrough  TsampIntegralVariant=Passthrough  ExternalSaturationOutDataTypeStr=Inherit: Same as second input
  Saturation1 : Saturate  UpperLimit=1  LowerLimit=0
  Saturation2 : Saturate  UpperLimit=1  LowerLimit=0
  Saturation3 : Saturate  UpperLimit=1  LowerLimit=0
  Sum : Sum  Inputs=|+-
  Sum1 : Sum  Inputs=|++
  Switch2 : Switch  Criteria=u2 > Threshold  Threshold=0.5  SaturateOnIntegerOverflow=off  InputSameDT=off
  y : Outport
  wires:
  Soll/1 -> Saturation1/1
  Saturation1/1 -> Sum/1
  Saturation2/1 -> Sum/2  "Sollgröße vor Regler"
  Constant/1 -> Sum1/2
  Saturation3/1 -> y/1
  Sum1/1 -> Saturation3/1
  PID Controller/1 -> Gain/1  "Stellgröße nach PID"
  1-D Lookup Table4/1 -> Sum1/1  "Stellgröße nach Offset"
  Constant5/1 -> PID Controller/3
  Constant1/1 -> PID Controller/2
  Freigabe/1 -> Switch2/2, PID Controller/4
  Switch2/1 -> PID Controller/1  "Regelabweichung"
  Sum/1 -> Switch2/1
  Constant6/1 -> Switch2/3
  Gain1/1 -> Saturation2/1
  "Ist "/1 -> Gain1/1
  Gain/1 -> 1-D Lookup Table4/1

== system D_20231120_Modell_Inbetriebnahme_BreakOutBox_Jetson/Lenkung Steuerung/Subsystem1 ==
  In1 : Inport
  1-D Lookup Table1 : Lookup_n-D  NumberOfTableDimensions=1  BreakpointsForDimension1=[0, 0.25,0.5,0.75 ,1]  Table=[0,0.40,0.5,0.60 ,1]  InternalRulePriority=Speed  RndMeth=Simplest
  Saturation : Saturate  UpperLimit=1  LowerLimit=0
  RC_LenkwinkelSoll : Outport
  wires:
  Saturation/1 -> 1-D Lookup Table1/1  "RC_LenkwinkelEingang"
  1-D Lookup Table1/1 -> RC_LenkwinkelSoll/1  "RC_LenkwinkelVorgabe"
  In1/1 -> Saturation/1

== system D_20231120_Modell_Inbetriebnahme_BreakOutBox_Jetson/Nvidia_Jetson/LaneFollowingAndControl ==
  Set velocity : Inport
  Longitudinal_Velocity : Inport  Port=2
  Lane Detections : Inport  Port=3
  Estimate Lane Center1 : Subsystem  VariantControl=v2
  MPC Controller : Subsystem
  steering_angle : Outport
  acceleration : Outport  Port=2
  wires:
  Longitudinal_Velocity/1 -> MPC Controller/2(Longitudinal velocity), Estimate Lane Center1/2(Longitudinal Velocity)
  MPC Controller/2(Acceleration) -> acceleration/1  "acceleration"
  Estimate Lane Center1/2(Lateral Offset) -> MPC Controller/4(Lateral deviation)  "lateral_deviation"
  Estimate Lane Center1/1(Previewed Curvature) -> MPC Controller/3(Curvature)  "previewed_curvature"
  Estimate Lane Center1/3(Heading Angle) -> MPC Controller/5(Relative yaw angle)  "relative_yaw_angle"
  Set velocity/1 -> MPC Controller/1(Set velocity)
  MPC Controller/1(Steering Angle) -> steering_angle/1  "steering_angle"
  Lane Detections/1 -> Estimate Lane Center1/1(Lane Detections)

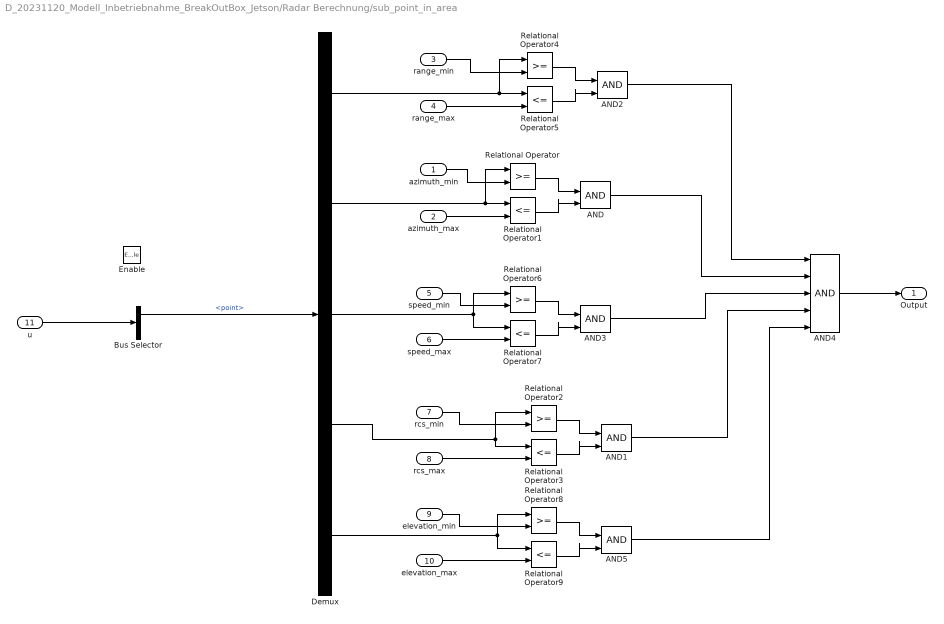
== system D_20231120_Modell_Inbetriebnahme_BreakOutBox_Jetson/Radar Berechnung/sub_point_in_area ==
  azimuth_min : Inport
  azimuth_max : Inport  Port=2
  range_min : Inport  Port=3
  range_max : Inport  Port=4
  speed_min : Inport  Port=5
  speed_max : Inport  Port=6
  rcs_min : Inport  Port=7
  rcs_max : Inport  Port=8
  elevation_min : Inport  Port=9
  elevation_max : Inport  Port=10
  u : Inport  Port=11
  Enable : EnablePort
  AND{,1..3,5} (5 alike) : Logic  IconShape=distinctive  AllPortsSameDT=off  OutDataTypeStr=boolean
  AND4 : Logic  Inputs=5  IconShape=distinctive  AllPortsSameDT=off  OutDataTypeStr=boolean
  Bus Selector : BusSelector  OutputSignals=point,CANID
  Demux : Demux  Outputs=5
  Relational Operator{,2,4,6,8} (5 alike) : RelationalOperator  OutDataTypeStr=boolean  RndMeth=Simplest  InputSameDT=off
  Relational Operator{1,3,5,7,9} (5 alike) : RelationalOperator  Operator=<=  OutDataTypeStr=boolean  RndMeth=Simplest  InputSameDT=off
  Output : Outport
  wires:
  Demux/5 -> Relational Operator8/1, Relational Operator9/1
  Demux/4 -> Relational Operator3/1, Relational Operator2/1
  Demux/3 -> Relational Operator6/1, Relational Operator7/1
  Demux/1 -> Relational Operator5/1, Relational Operator4/1
  Demux/2 -> Relational Operator1/1, Relational Operator/1
  elevation_max/1 -> Relational Operator9/2
  AND5/1 -> AND4/5
  Relational Operator8/1 -> AND5/1
  Relational Operator9/1 -> AND5/2
  elevation_min/1 -> Relational Operator8/2
  range_min/1 -> Relational Operator4/2
  azimuth_min/1 -> Relational Operator/2
  speed_min/1 -> Relational Operator6/2
  rcs_min/1 -> Relational Operator2/2
  Relational Operator6/1 -> AND3/1
  Relational Operator/1 -> AND/1
  AND4/1 -> Output/1
  Relational Operator4/1 -> AND2/1
  Relational Operator2/1 -> AND1/1
  Relational Operator5/1 -> AND2/2
  Relational Operator3/1 -> AND1/2
  Relational Operator7/1 -> AND3/2
  speed_max/1 -> Relational Operator7/2
  Relational Operator1/1 -> AND/2
  AND2/1 -> AND4/1
  u/1 -> Bus Selector/1
  AND/1 -> AND4/2
  AND1/1 -> AND4/4
  Bus Selector/1 -> Demux/1  "<point>"
  rcs_max/1 -> Relational Operator3/2
  range_max/1 -> Relational Operator5/2
  AND3/1 -> AND4/3
  azimuth_max/1 -> Relational Operator1/2

== system D_20231120_Modell_Inbetriebnahme_BreakOutBox_Jetson/Bremspedal Steuerung/QAD Steuerung1/Anti-Relaisprellen ==
  In : Inport
  Bias : Bias  Bias=-Ts  SaturateOnIntegerOverflow=off
  Compare To Zero : simulink/Logic and Bit Operations/Compare To Zero  relop===  OutDataTypeStr=boolean
  Constant : Constant  Value=0.01
  Constant1 : Constant  Value=0
  Delay1 : Delay  DelayLength=1  InputProcessing=Columns as channels (frame based)
  Detect Increase : simulink/Logic and Bit Operations/Detect Increase  vinit=0.0  OutDataTypeStr=boolean
  Saturation : Saturate  UpperLimit=0.2  LowerLimit=0
  Switch : Switch  Criteria=u2 ~= 0  SaturateOnIntegerOverflow=off  InputSameDT=off
  Switch1 : Switch  Criteria=u2 ~= 0  SaturateOnIntegerOverflow=off  InputSameDT=off
  Out : Outport  VectorParamsAs1DForOutWhenUnconnected=off
  wires:
  Compare To Zero/1 -> Switch1/2
  In/1 -> Detect Increase/1, Switch1/1
  Switch1/1 -> Out/1
  Constant1/1 -> Switch1/3
  Delay1/1 -> Bias/1, Compare To Zero/1
  Constant/1 -> Switch/1
  Detect Increase/1 -> Switch/2
  Switch/1 -> Delay1/1
  Bias/1 -> Saturation/1
  Saturation/1 -> Switch/3

== system D_20231120_Modell_Inbetriebnahme_BreakOutBox_Jetson/Bremspedal Steuerung/QAD Steuerung1/Anti-Relaisprellen1 ==
  In : Inport
  Bias : Bias  Bias=-Ts  SaturateOnIntegerOverflow=off
  Compare To Zero : simulink/Logic and Bit Operations/Compare To Zero  relop===  OutDataTypeStr=boolean
  Constant : Constant  Value=0.01  VectorParams1D=off
  Constant1 : Constant  Value=0
  Delay1 : Delay  DelayLength=1  InputProcessing=Columns as channels (frame based)
  Detect Increase : simulink/Logic and Bit Operations/Detect Increase  vinit=0.0  OutDataTypeStr=boolean
  Saturation : Saturate  UpperLimit=0.2  LowerLimit=0
  Switch : Switch  Criteria=u2 ~= 0  SaturateOnIntegerOverflow=off  InputSameDT=off
  Switch1 : Switch  Criteria=u2 ~= 0  SaturateOnIntegerOverflow=off  InputSameDT=off
  Out : Outport  VectorParamsAs1DForOutWhenUnconnected=off
  wires:
  Compare To Zero/1 -> Switch1/2
  In/1 -> Detect Increase/1, Switch1/1
  Switch1/1 -> Out/1
  Constant1/1 -> Switch1/3
  Delay1/1 -> Bias/1, Compare To Zero/1
  Constant/1 -> Switch/1
  Detect Increase/1 -> Switch/2
  Switch/1 -> Delay1/1
  Bias/1 -> Saturation/1
  Saturation/1 -> Switch/3

== system D_20231120_Modell_Inbetriebnahme_BreakOutBox_Jetson/Bremspedal Steuerung/QAD Steuerung1/Counter ==
  count_dir : Inport
  count_enable : Inport  Port=2
  count_reset : Inport  Port=3
  AND5 : Logic  AllPortsSameDT=off  OutDataTypeStr=boolean
  AND6 : Logic  AllPortsSameDT=off  OutDataTypeStr=boolean
  Add : Sum
  Compare To Constant5 : simulink/Logic and Bit Operations/Compare To Constant  relop===  const=1  OutDataTypeStr=boolean
  Compare To Zero : simulink/Logic and Bit Operations/Compare To Zero  relop=>  OutDataTypeStr=boolean
  Compare To Zero1 : simulink/Logic and Bit Operations/Compare To Zero  relop===  OutDataTypeStr=boolean
  Constant : Constant  Value=-1
  Constant1 : Constant  Value=0
  Constant2 : Constant
  Constant3 : Constant  Value=0
  Switch : Switch  Criteria=u2 > Threshold  SaturateOnIntegerOverflow=off  InputSameDT=off
  Switch1 : Switch  Criteria=u2 > Threshold  SaturateOnIntegerOverflow=off  InputSameDT=off
  Switch2 : Switch  Criteria=u2 > Threshold  Threshold=0.5  SaturateOnIntegerOverflow=off  InputSameDT=off
  Unit Delay : UnitDelay  SampleTime=-1  HasFrameUpgradeWarning=on
  Unit Delay1 : UnitDelay  SampleTime=-1  HasFrameUpgradeWarning=on
  Value : Outport
  wires:
  count_dir/1 -> Compare To Zero1/1, Compare To Constant5/1
  Compare To Zero/1 -> AND6/2, AND5/2
  Constant1/1 -> Switch/3
  AND6/1 -> Switch1/2
  Switch1/1 -> Add/1
  AND5/1 -> Switch/2
  Switch/1 -> Switch1/3
  Compare To Constant5/1 -> AND5/1
  Constant2/1 -> Switch1/1
  Compare To Zero1/1 -> AND6/1
  Constant/1 -> Switch/1
  count_enable/1 -> Compare To Zero/1
  Add/1 -> Unit Delay/1, Value/1
  count_reset/1 -> Unit Delay1/1
  Constant3/1 -> Switch2/1
  Switch2/1 -> Add/2
  Unit Delay1/1 -> Switch2/2
  Unit Delay/1 -> Switch2/3

== system D_20231120_Modell_Inbetriebnahme_BreakOutBox_Jetson/Bremspedal Steuerung/QAD Steuerung1/QAD1 ==
  Hall_A : Inport
  Hall_B : Inport  Port=2
  Data Type Conversion : DataTypeConversion  SaturateOnIntegerOverflow=off  RndMeth=Floor
  Data Type Conversion1 : DataTypeConversion  SaturateOnIntegerOverflow=off  RndMeth=Floor
  State Transition Table : State Transition Table  TreatAsAtomicUnit=on
  Count_direction : Outport
  Count_enable : Outport  Port=2
  wires:
  Hall_A/1 -> Data Type Conversion/1
  Hall_B/1 -> Data Type Conversion1/1
  Data Type Conversion/1 -> State Transition Table/1(Hall_A)
  Data Type Conversion1/1 -> State Transition Table/2(Hall_B)
  State Transition Table/1(count_enable) -> Count_enable/1
  State Transition Table/2(count_dir) -> Count_direction/1

== system D_20231120_Modell_Inbetriebnahme_BreakOutBox_Jetson/Freigabe/Freigabe/1s Tastersperre ==
  In : Inport
  Bias : Bias  Bias=-Ts  SaturateOnIntegerOverflow=off
  Compare To Zero : simulink/Logic and Bit Operations/Compare To Zero  relop===  OutDataTypeStr=boolean
  Constant : Constant
  Constant1 : Constant  Value=0
  Delay1 : Delay  DelayLength=1  InputProcessing=Columns as channels (frame based)
  Detect Increase : simulink/Logic and Bit Operations/Detect Increase  vinit=0.0  OutDataTypeStr=boolean
  Saturation : Saturate  UpperLimit=1  LowerLimit=0
  Switch : Switch  Criteria=u2 ~= 0  SaturateOnIntegerOverflow=off  InputSameDT=off
  Switch1 : Switch  Criteria=u2 ~= 0  SaturateOnIntegerOverflow=off  InputSameDT=off
  Out : Outport  VectorParamsAs1DForOutWhenUnconnected=off
  wires:
  Compare To Zero/1 -> Switch1/2
  In/1 -> Detect Increase/1, Switch1/1
  Switch1/1 -> Out/1
  Constant1/1 -> Switch1/3
  Delay1/1 -> Bias/1, Compare To Zero/1
  Constant/1 -> Switch/1
  Detect Increase/1 -> Switch/2
  Switch/1 -> Delay1/1
  Bias/1 -> Saturation/1
  Saturation/1 -> Switch/3

== system D_20231120_Modell_Inbetriebnahme_BreakOutBox_Jetson/Freigabe/Freigabe/Detektion Fahrpedal ==
  FP_1_In : Inport
  FP_2_In : Inport  Port=2
  AND : Logic  AllPortsSameDT=off  OutDataTypeStr=boolean
  Compare To Constant : simulink/Logic and Bit Operations/Compare To Constant  relop=<=  const=1.1  OutDataTypeStr=boolean
  Compare To Constant1 : simulink/Logic and Bit Operations/Compare To Constant  relop=<=  const=0.7  OutDataTypeStr=boolean
  Moving Average : Subsystem
  Moving Average1 : Subsystem
  FP_Freigabe : Outport
  wires:
  FP_1_In/1 -> Moving Average/1(In)
  FP_2_In/1 -> Moving Average1/1(In)
  AND/1 -> FP_Freigabe/1
  Moving Average/1(Out) -> Compare To Constant/1
  Moving Average1/1(Out) -> Compare To Constant1/1
  Compare To Constant/1 -> AND/1
  Compare To Constant1/1 -> AND/2
